simulink model "motor_model_asama1"  (R2026a)
settings: Solver=VariableStepAuto  StopTime=5
settings Model: Creator=alpagumagus  LastModifiedBy=alpagumagus

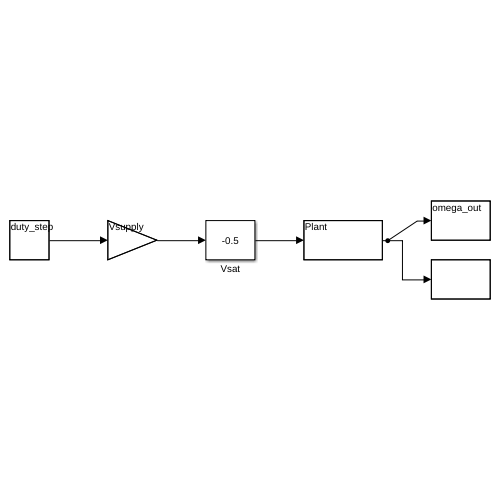
[thumbnail: Simulink's stored preview of the top-level diagram]
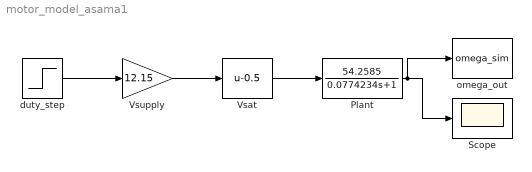
== system motor_model_asama1 ==
  Plant : TransferFcn  Numerator=[54.2585]  Denominator=[0.0774234 1]
  Scope : Scope
  Vsat : Bias  Bias=-0.5  SaturateOnIntegerOverflow=off
  Vsupply : Gain  Gain=12.15
  duty_step : Step  Time=0  FinalValue=0.30  SampleTime=0
  omega_out : ToWorkspace  VariableName=omega_sim  SaveFormat=Timeseries  SampleTime=-1
  wires:
  duty_step/1 -> Vsupply/1
  Vsupply/1 -> Vsat/1
  Vsat/1 -> Plant/1
  Plant/1 -> omega_out/1, Scope/1
